simulink model "pendulumSystem"  (R2023b)
settings: Solver=VariableStepAuto  StartTime=0.0  StopTime=10.0  RelTol=1e-3
undefined symbols (not defined in the file or in its folder): X, Y, Z
libraries: sm_lib x8, nesl_utility x6, simulink_extras x3, fuzblock x2, slpidlib x2, simulink x1
settings Model: Creator=allef  LastModifiedBy=allef
settings SolverCC: ZeroCrossControl=DisableAll

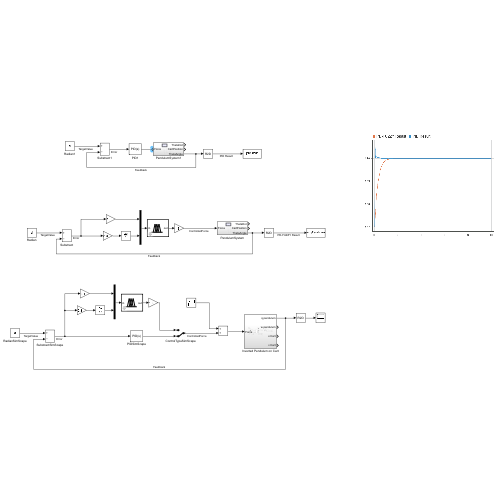
[thumbnail: Simulink's stored preview of the top-level diagram]
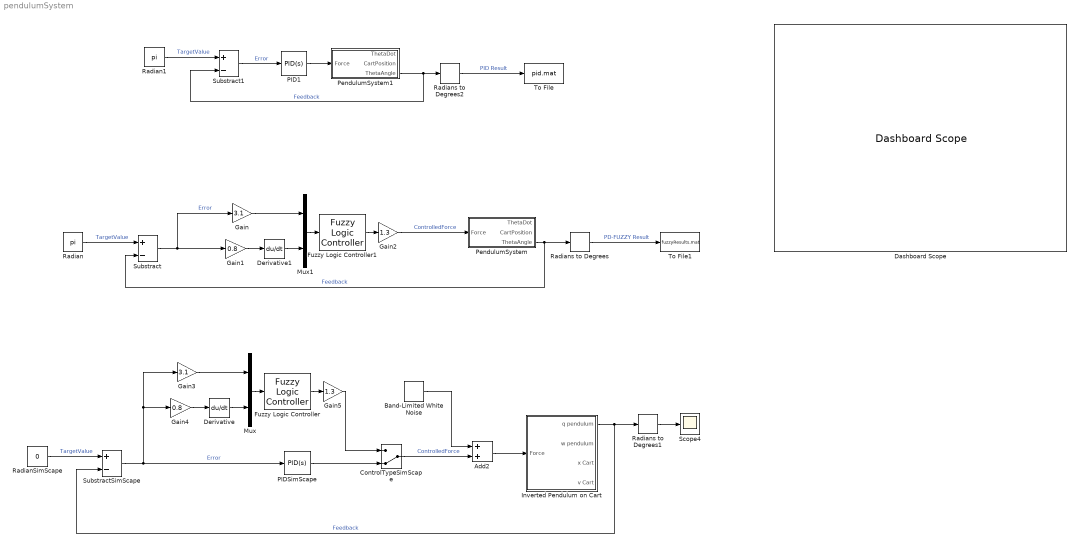
== system pendulumSystem ==
  Add2 : Sum
  Band-Limited White Noise : simulink/Sources/Band-Limited White Noise  Cov=[0.01]  Ts=0.1  seed=[23341]
  ControlTypeSimScape : ManualSwitch  CurrentSetting=0
  Dashboard Scope : DashboardScope
  Derivative : Derivative
  Derivative1 : Derivative
  Fuzzy Logic Controller : fuzblock/Fuzzy Logic  Controller  FIS='Fuzzy.fis'  OutputSampleNumber=101  DataType=double  FuzzifiedInputs=off  RuleFiringStrengths=off  RuleOutputs=off  AggregatedOutputs=off  SimulateUsing=Interpreted execution  OutOfRangeInputValueMessage=warning  NoRuleFiredMessage=warning  EmptyOutputFuzzySetMessage=warning
  Fuzzy Logic Controller1 : fuzblock/Fuzzy Logic  Controller  FIS='Fuzzy.fis'  OutputSampleNumber=101  DataType=double  FuzzifiedInputs=off  RuleFiringStrengths=off  RuleOutputs=off  AggregatedOutputs=off  SimulateUsing=Interpreted execution  OutOfRangeInputValueMessage=warning  NoRuleFiredMessage=warning  EmptyOutputFuzzySetMessage=warning
  Gain : Gain  Gain=3.1
  Gain1 : Gain  Gain=0.8
  Gain2 : Gain  Gain=1.3
  Gain3 : Gain  Gain=3.1
  Gain4 : Gain  Gain=0.8
  Gain5 : Gain  Gain=1.3
  Inverted Pendulum on Cart : Subsystem
  Mux : Mux  Inputs=2
  Mux1 : Mux  Inputs=2
  PID1 : slpidlib/PID Controller  Controller=PID  Form=Parallel  TimeDomain=Continuous-time  UseExternalTs=off  SampleTime=-1  IntegratorMethod=Forward Euler  FilterMethod=Forward Euler  ControllerParametersSource=internal  P=100  I=1  UseKiTs=off  D=20  N=100  UseFilter=on  TunerSelectOption=Transfer Function Based (PID Tuner App)  InitialConditionSource=internal  InitialConditionForIntegrator=0  InitialConditionForFilter=0  DifferentiatorICPrevScaledInput=0  ExternalReset=none  TrackingMode=off  Kt=1  LimitOutput=off  SatLimitsSource=internal  UpperSaturationLimit=inf  LowerSaturationLimit=-inf  LinearizeAsGain=on  AntiWindupMode=none  Kb=1  LimitIntegrator=off  UpperIntegratorSaturationLimit=inf  LowerIntegratorSaturationLimit=-inf  POutMin=[]  POutMax=[]  IOutMin=[]  IOutMax=[]  DOutMin=[]  DOutMax=[]  NOutMin=[]  NOutMax=[]  SumOutMin=[]  SumOutMax=[]  SaturationOutMin=[]  SaturationOutMax=[]  PParamMin=[]  PParamMax=[]  IParamMin=[]  IParamMax=[]  DParamMin=[]  DParamMax=[]  NParamMin=[]  NParamMax=[]  KbParamMin=[]  KbParamMax=[]  KtParamMin=[]  KtParamMax=[]  KbOutMin=[]  KbOutMax=[]  KtOutMin=[]  KtOutMax=[]  IntegratorOutMin=[]  IntegratorOutMax=[]  FilterOutMin=[]  FilterOutMax=[]  SumI1OutMin=[]  SumI1OutMax=[]  SumI2OutMin=[]  SumI2OutMax=[]  SumI3OutMin=[]  SumI3OutMax=[]  SumI4OutMin=[]  SumI4OutMax=[]  SumDOutMin=[]  SumDOutMax=[]  DifferentiatorOutMin=[]  DifferentiatorOutMax=[]  FilterDiffOutCoefMin=[]  FilterDiffOutCoefMax=[]  ReciprocalOutMin=[]  ReciprocalOutMax=[]  SumDenOutMin=[]  SumDenOutMax=[]  SumNumOutMin=[]  SumNumOutMax=[]  DivideOutMin=[]  DivideOutMax=[]  UdiffTsProdOutMin=[]  UdiffTsProdOutMax=[]  NTsProdOutMin=[]  NTsProdOutMax=[]  UintegralTsProdOutMin=[]  UintegralTsProdOutMax=[]  UngainTsProdOutMin=[]  UngainTsProdOutMax=[]  ClampingZeroOutDataTypeStr=Inherit: Inherit via back propagation  ClampingZeroOutMin=[]  ClampingZeroOutMax=[]  FilterDenConstantOutDataTypeStr=Inherit: Inherit via back propagation  FilterDenConstantOutMin=[]  FilterDenConstantOutMax=[]  PCopyOutDataTypeStr=Inherit: Inherit via back propagation  PCopyOutMin=[]  PCopyOutMax=[]  NCopyOutDataTypeStr=Inherit: Inherit via back propagation  NCopyOutMin=[]  NCopyOutMax=[]  IntegratorContinuousStateAttributes=''  IntegratorStateMustResolveToSignalObject=off  IntegratorRTWStateStorageClass=Auto  FilterContinuousStateAttributes=''  FilterStateMustResolveToSignalObject=off  FilterRTWStateStorageClass=Auto  ParallelPVariant=InternalParameters  IdealPVariant=Disabled  IVariant=InternalParameters  DVariant=InternalParameters  IntegratorVariant=Continuous  SatVariant=Disabled  AWVariant=Passthrough  PCopyVariant=Disabled  TRVariant=Disabled  FdbkBlocksVariant=Forward  IdealPFdbkVariant=Disabled  SatFdbkVariant=Disabled  DerivativeFilterVariant=ContFilter  NVariant=InternalParameters  NCopyVariant=Disabled  FilterICVariant=InternalICsFilter  IntegratorICVariant=InternalICs  ExternalResetVariant=Disabled  TRSumVariant=Passthrough  SumFdbkVariant=Disabled  SumVariant=Sum_PID  TsampFilterVariant=InternalTs  TsampNgainVariant=Passthrough  TsampIntegralVariant=Disabled_SignalSpec  ExternalSaturationOutDataTypeStr=Inherit: Same as second input
  PIDSimScape : slpidlib/PID Controller  Controller=PID  Form=Parallel  TimeDomain=Continuous-time  UseExternalTs=off  SampleTime=-1  IntegratorMethod=Forward Euler  FilterMethod=Forward Euler  ControllerParametersSource=internal  P=100  I=1  UseKiTs=off  D=20  N=100  UseFilter=on  TunerSelectOption=Transfer Function Based (PID Tuner App)  InitialConditionSource=internal  InitialConditionForIntegrator=0  InitialConditionForFilter=0  DifferentiatorICPrevScaledInput=0  ExternalReset=none  TrackingMode=off  Kt=1  LimitOutput=off  SatLimitsSource=internal  UpperSaturationLimit=inf  LowerSaturationLimit=-inf  LinearizeAsGain=on  AntiWindupMode=none  Kb=1  LimitIntegrator=off  UpperIntegratorSaturationLimit=inf  LowerIntegratorSaturationLimit=-inf  POutMin=[]  POutMax=[]  IOutMin=[]  IOutMax=[]  DOutMin=[]  DOutMax=[]  NOutMin=[]  NOutMax=[]  SumOutMin=[]  SumOutMax=[]  SaturationOutMin=[]  SaturationOutMax=[]  PParamMin=[]  PParamMax=[]  IParamMin=[]  IParamMax=[]  DParamMin=[]  DParamMax=[]  NParamMin=[]  NParamMax=[]  KbParamMin=[]  KbParamMax=[]  KtParamMin=[]  KtParamMax=[]  KbOutMin=[]  KbOutMax=[]  KtOutMin=[]  KtOutMax=[]  IntegratorOutMin=[]  IntegratorOutMax=[]  FilterOutMin=[]  FilterOutMax=[]  SumI1OutMin=[]  SumI1OutMax=[]  SumI2OutMin=[]  SumI2OutMax=[]  SumI3OutMin=[]  SumI3OutMax=[]  SumI4OutMin=[]  SumI4OutMax=[]  SumDOutMin=[]  SumDOutMax=[]  DifferentiatorOutMin=[]  DifferentiatorOutMax=[]  FilterDiffOutCoefMin=[]  FilterDiffOutCoefMax=[]  ReciprocalOutMin=[]  ReciprocalOutMax=[]  SumDenOutMin=[]  SumDenOutMax=[]  SumNumOutMin=[]  SumNumOutMax=[]  DivideOutMin=[]  DivideOutMax=[]  UdiffTsProdOutMin=[]  UdiffTsProdOutMax=[]  NTsProdOutMin=[]  NTsProdOutMax=[]  UintegralTsProdOutMin=[]  UintegralTsProdOutMax=[]  UngainTsProdOutMin=[]  UngainTsProdOutMax=[]  ClampingZeroOutDataTypeStr=Inherit: Inherit via back propagation  ClampingZeroOutMin=[]  ClampingZeroOutMax=[]  FilterDenConstantOutDataTypeStr=Inherit: Inherit via back propagation  FilterDenConstantOutMin=[]  FilterDenConstantOutMax=[]  PCopyOutDataTypeStr=Inherit: Inherit via back propagation  PCopyOutMin=[]  PCopyOutMax=[]  NCopyOutDataTypeStr=Inherit: Inherit via back propagation  NCopyOutMin=[]  NCopyOutMax=[]  IntegratorContinuousStateAttributes=''  IntegratorStateMustResolveToSignalObject=off  IntegratorRTWStateStorageClass=Auto  FilterContinuousStateAttributes=''  FilterStateMustResolveToSignalObject=off  FilterRTWStateStorageClass=Auto  ParallelPVariant=InternalParameters  IdealPVariant=Disabled  IVariant=InternalParameters  DVariant=InternalParameters  IntegratorVariant=Continuous  SatVariant=Disabled  AWVariant=Passthrough  PCopyVariant=Disabled  TRVariant=Disabled  FdbkBlocksVariant=Forward  IdealPFdbkVariant=Disabled  SatFdbkVariant=Disabled  DerivativeFilterVariant=ContFilter  NVariant=InternalParameters  NCopyVariant=Disabled  FilterICVariant=InternalICsFilter  IntegratorICVariant=InternalICs  ExternalResetVariant=Disabled  TRSumVariant=Passthrough  SumFdbkVariant=Disabled  SumVariant=Sum_PID  TsampFilterVariant=InternalTs  TsampNgainVariant=Passthrough  TsampIntegralVariant=Disabled_SignalSpec  ExternalSaturationOutDataTypeStr=Inherit: Same as second input
  PendulumSystem : Subsystem
  PendulumSystem1 : Subsystem
  Radian : Constant  Value=pi
  Radian1 : Constant  Value=pi
  RadianSimScape : Constant  Value=0
  Radians to Degrees : simulink_extras/Transformations/Radians to Degrees
  Radians to Degrees1 : simulink_extras/Transformations/Radians to Degrees
  Radians to Degrees2 : simulink_extras/Transformations/Radians to Degrees
  Scope4 : Scope
  Substract : Sum  Inputs=+-
  Substract1 : Sum  Inputs=+-
  SubstractSimScape : Sum  Inputs=+-
  To File : ToFile  Filename=pid.mat  MatrixName=pid
  To File1 : ToFile  Filename=fuzzyResults.mat  MatrixName=fuzzy
  wires:
  Substract/1 -> Gain/1, Gain1/1  "Error"
  Radian/1 -> Substract/1  "TargetValue"
  PendulumSystem/3(ThetaAngle) -> Substract/2, Radians to Degrees/1  "Feedback"
  Radians to Degrees/1 -> To File1/1  "PD-FUZZY Result"
  ControlTypeSimScape/1 -> Add2/2  "ControlledForce"
  RadianSimScape/1 -> SubstractSimScape/1  "TargetValue"
  SubstractSimScape/1 -> PIDSimScape/1, Gain4/1, Gain3/1  "Error"
  PIDSimScape/1 -> ControlTypeSimScape/2
  Derivative/1 -> Mux/2
  Mux/1 -> Fuzzy Logic Controller/1
  Fuzzy Logic Controller/1 -> Gain5/1
  Derivative1/1 -> Mux1/2
  Mux1/1 -> Fuzzy Logic Controller1/1
  Fuzzy Logic Controller1/1 -> Gain2/1
  Gain/1 -> Mux1/1
  Gain1/1 -> Derivative1/1
  Gain3/1 -> Mux/1
  Gain4/1 -> Derivative/1
  Gain5/1 -> ControlTypeSimScape/1
  Add2/1 -> Inverted Pendulum on Cart/1(Force)
  Inverted Pendulum on Cart/1(q pendulum) -> SubstractSimScape/2, Radians to Degrees1/1  "Feedback"
  Radians to Degrees1/1 -> Scope4/1
  Gain2/1 -> PendulumSystem/1(Force)  "ControlledForce"
  Band-Limited White Noise/1 -> Add2/1
  Radians to Degrees2/1 -> To File/1  "PID Result"
  PendulumSystem1/3(ThetaAngle) -> Radians to Degrees2/1, Substract1/2  "Feedback"
  PID1/1 -> PendulumSystem1/1(Force)
  Radian1/1 -> Substract1/1  "TargetValue"
  Substract1/1 -> PID1/1  "Error"

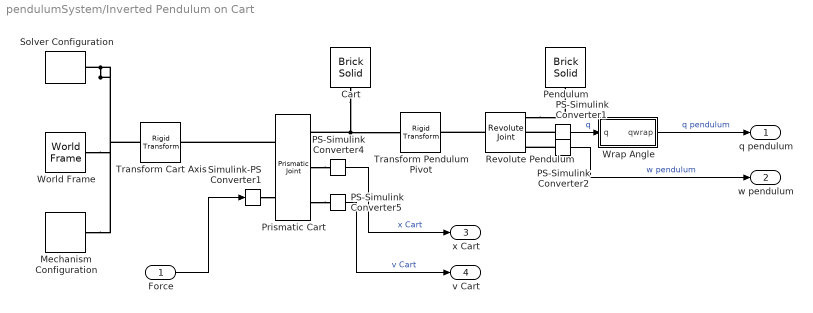
== system pendulumSystem/Inverted Pendulum on Cart ==
  Force : Inport
  Cart : sm_lib/Body Elements/Brick Solid  GraphicAmbientColor=[0.15 0.15 0.15 1.0]  BasedOnType=Density  BrickDimensions=[0.2 0.04 .60]  BrickDimensionsUnits=m  CenterOfMass=[0 0 0]  CenterOfMassUnits=m  GraphicDiffuseColor=[0.8 0.45 0]  Density=1000  DensityUnits=kg/m^3  DoExposeReferenceFrame=on  GraphicEmissiveColor=[0.0 0.0 0.0 1.0]  ExportEntireGeometry=off  SerializedFrames=<Frames/>  MarkerShape=Sphere  MarkerSize=10  GraphicType=FromGeometry  InertiaType=PointMass  Mass=0.5  MassUnits=kg  MomentsOfInertia=[1 1 1]  MomentsOfInertiaUnits=kg*m^2  GraphicOpacity=1.0  ProductsOfInertia=[0 0 0]  ProductsOfInertiaUnits=kg*m^2  GraphicShininess=75  GraphicSpecularColor=[0.5 0.5 0.5 1.0]  GraphicVisPropType=SimpleVisualProperties
  Mechanism Configuration : sm_lib/Utilities/Mechanism Configuration  UniformGravity=Constant  GravityVector=[0 0 -9.80665]  GravityVectorUnits=m/s^2  LinearizationDelta=0.001  JointModeTransitionNonlinearIterations=2
  PS-Simulink Converter1 : nesl_utility/PS-Simulink Converter  PhysicalDomain=network_engine_domain  SubClassName=ps_output  LeftPortType=input  RightPortType=output  PseudoPeriodic=off  Frequencies=[]  VectorFormat=1-D array  Unit=rad  AffineConversion=off
  PS-Simulink Converter2 : nesl_utility/PS-Simulink Converter  PhysicalDomain=network_engine_domain  SubClassName=ps_output  LeftPortType=input  RightPortType=output  PseudoPeriodic=off  Frequencies=[]  VectorFormat=1-D array  Unit=rad/s  AffineConversion=off
  PS-Simulink Converter4 : nesl_utility/PS-Simulink Converter  PhysicalDomain=network_engine_domain  SubClassName=ps_output  LeftPortType=input  RightPortType=output  PseudoPeriodic=off  Frequencies=[]  VectorFormat=1-D array  Unit=m  AffineConversion=off
  PS-Simulink Converter5 : nesl_utility/PS-Simulink Converter  PhysicalDomain=network_engine_domain  SubClassName=ps_output  LeftPortType=input  RightPortType=output  PseudoPeriodic=off  Frequencies=[]  VectorFormat=1-D array  Unit=m/s  AffineConversion=off
  Pendulum : sm_lib/Body Elements/Brick Solid  GraphicAmbientColor=[0.15 0.15 0.15 1.0]  BasedOnType=Density  BrickDimensions=[0.6 0.03 0.05]  BrickDimensionsUnits=m  CenterOfMass=[0 0 0]  CenterOfMassUnits=m  GraphicDiffuseColor=[0.25 0.4 0.7]  Density=1000  DensityUnits=kg/m^3  DoExposeReferenceFrame=off  GraphicEmissiveColor=[0.0 0.0 0.0 1.0]  ExportEntireGeometry=off  SerializedFrames=<Frames><Frame><Id>Frame1</Id><Value><Name>B</Name><Origin><Source>GeometricFeature</Source><FeatureName>+x surface</FeatureName></Origin><PrimaryAxis><DefinedDirection>+Z</DefinedDirection><Source>ReferenceFrame</Source><SourceDirection>+Z</SourceDirection><FeatureName></FeatureName></PrimaryAxis><SecondaryAxis><DefinedDirection>+X</DefinedDirection><Source>ReferenceFrame</Source><SourceDirection>+X</SourceDirection><FeatureName></FeatureName></SecondaryAxis></Value></Frame></Frames>  MarkerShape=Sphere  MarkerSize=10  GraphicType=FromGeometry  InertiaType=PointMass  Mass=0.2  MassUnits=kg  MomentsOfInertia=[1 1 1]  MomentsOfInertiaUnits=kg*m^2  GraphicOpacity=1.0  ProductsOfInertia=[0 0 0]  ProductsOfInertiaUnits=kg*m^2  GraphicShininess=75  GraphicSpecularColor=[0.5 0.5 0.5 1.0]  GraphicVisPropType=SimpleVisualProperties
  Prismatic Cart : sm_lib/Joints/Prismatic Joint  JointMode=Normal  SenseConstraintForce=off  SenseConstraintForceX=off  SenseConstraintForceY=off  SenseConstraintForceZ=off  SenseConstraintTorque=off  SenseConstraintTorqueX=off  SenseConstraintTorqueY=off  SenseConstraintTorqueZ=off  SenseTotalForce=off  SenseTotalForceX=off  SenseTotalForceY=off  SenseTotalForceZ=off  SenseTotalTorque=off  SenseTotalTorqueX=off  SenseTotalTorqueY=off  SenseTotalTorqueZ=off  CompositeWrenchDir=FollowerOnBase  CompositeWrenchFrame=BaseFrame  EquilibriumPosition=0  EquilibriumPositionUnits=m  SpringStiffness=0  SpringStiffnessUnits=N/m  DampingCoefficient=0.1  DampingCoefficientUnits=N/(m/s)  TorqueActuationMode=InputTorque  MotionActuationMode=ComputedMotion  SensePosition=on  SenseVelocity=on  SenseAcceleration=off  SenseTorqueForce=off  SenseLowerLimitTorqueForce=off  SenseUpperLimitTorqueForce=off  LowerLimitSpecify=off  LowerLimitBound=-1  LowerLimitBoundUnits=m  LowerLimitStiffness=1e6  LowerLimitStiffnessUnits=N/m  LowerLimitDamping=1e3  LowerLimitDampingUnits=N/(m/s)  LowerLimitTransitionRegionWidth=1e-4  LowerLimitTransitionRegionWidthUnits=m  UpperLimitSpecify=off  UpperLimitBound=1  UpperLimitBoundUnits=m  UpperLimitStiffness=1e6  UpperLimitStiffnessUnits=N/m  UpperLimitDamping=1e3  UpperLimitDampingUnits=N/(m/s)  UpperLimitTransitionRegionWidth=1e-4  UpperLimitTransitionRegionWidthUnits=m  PositionTargetSpecify=off  PositionTargetPriority=High  PositionTargetValue=0  PositionTargetValueUnits=m  VelocityTargetSpecify=off  VelocityTargetPriority=High  VelocityTargetValue=0  VelocityTargetValueUnits=m/s
  Revolute Pendulum : sm_lib/Joints/Revolute Joint  JointMode=Normal  SenseConstraintForce=off  SenseConstraintForceX=off  SenseConstraintForceY=off  SenseConstraintForceZ=off  SenseConstraintTorque=off  SenseConstraintTorqueX=off  SenseConstraintTorqueY=off  SenseConstraintTorqueZ=off  SenseTotalForce=off  SenseTotalForceX=off  SenseTotalForceY=off  SenseTotalForceZ=off  SenseTotalTorque=off  SenseTotalTorqueX=off  SenseTotalTorqueY=off  SenseTotalTorqueZ=off  CompositeWrenchDir=FollowerOnBase  CompositeWrenchFrame=BaseFrame  EquilibriumPosition=0  EquilibriumPositionUnits=deg  SpringStiffness=0  SpringStiffnessUnits=N*m/deg  DampingCoefficient=0  DampingCoefficientUnits=N*m/(deg/s)  TorqueActuationMode=NoTorque  MotionActuationMode=ComputedMotion  SensePosition=on  SenseVelocity=on  SenseAcceleration=off  SenseTorqueForce=off  SenseLowerLimitTorqueForce=off  SenseUpperLimitTorqueForce=off  LowerLimitSpecify=off  LowerLimitBound=-90  LowerLimitBoundUnits=deg  LowerLimitStiffness=1e4  LowerLimitStiffnessUnits=N*m/deg  LowerLimitDamping=10  LowerLimitDampingUnits=N*m/(deg/s)  LowerLimitTransitionRegionWidth=0.1  LowerLimitTransitionRegionWidthUnits=deg  UpperLimitSpecify=off  UpperLimitBound=90  UpperLimitBoundUnits=deg  UpperLimitStiffness=1e4  UpperLimitStiffnessUnits=N*m/deg  UpperLimitDamping=10  UpperLimitDampingUnits=N*m/(deg/s)  UpperLimitTransitionRegionWidth=0.1  UpperLimitTransitionRegionWidthUnits=deg  PositionTargetSpecify=off  PositionTargetPriority=High  PositionTargetValue=0  PositionTargetValueUnits=deg  VelocityTargetSpecify=off  VelocityTargetPriority=High  VelocityTargetValue=0  VelocityTargetValueUnits=deg/s
  Simulink-PS Converter1 : nesl_utility/Simulink-PS Converter  PhysicalDomain=network_engine_domain  SubClassName=ps_input  LeftPortType=input  RightPortType=output  PseudoPeriodic=off  Frequencies=[]  NoiseDistribution=none  NoiseParameters=[]  Unit=N  AffineConversion=off  FilteringAndDerivatives=zero  SimscapeFilterOrder=1  InputFilterTimeConstant=.001  UdotUserProvided=1
  Solver Configuration : nesl_utility/Solver Configuration  PhysicalDomain=network_engine_domain  SubClassName=solver  LeftPortType=input  RightPortType=generic  Tones=[]  Harmonics=[]  SimulateNoise=off  Profile=off  UseLocalSampling=off  EnableSwitchedLinearOptims=on  FrequencyDomain=off  UseCCode=off  RelTol=0.001  AbsTol=1e-06  MinStep=1e-09  ToWorkspace=off  RevertToSquareIcSolve=off  NumHomotopyIterations=100  PhasorMode=off  PhasorModeNumHarmonics=1  ConsistencySolver=NEWTON_FTOL  IndexReductionMethod=DerivativeReplacement  DoDC=off  ResidualTolerance=1e-09  ConsistencyTolSource=GLOBAL  ConsistencyAbsTol=0.001  ConsistencyRelTol=0.001  ConsistencyTolFactor=0.001  UseLocalSolver=off  LocalSolverChoice=NE_BACKWARD_EULER_ADVANCER  ResolveIndetEquations=on  FunctionEvalNumThread=1  LocalSolverSampleTime=0.001  DoFixedCost=off  MaxNonlinIter=3  MaxModeIter=2  ComputeImpulses=off  ImpulseIterations=2  LinearAlgebra=Sparse  LinearAlgebraNumThread=0  EquationFormulation=NE_TIME_EF  DelaysMemoryBudget=1024  AutomaticFiltering=on  FilteringTimeConstant=0.001  PartitionStorageMethod=AS_NEEDED  PartitionMemoryBudget=1024  PartitionMethod=FAST  MultibodyUseLocalSolver=off  MultibodyLocalSolverChoice=ODE1  MultibodyLocalSolverSampleTime=0.001
  Transform Cart Axis : sm_lib/Frames and Transforms/Rigid Transform  TranslationMethod=None  TranslationStandardOffset=0  TranslationStandardOffsetUnits=m  TranslationStandardAxis=+Z  TranslationCartesianOffset=[0 0 0]  TranslationCartesianOffsetUnits=m  TranslationROffset=0  TranslationROffsetUnits=m  TranslationZOffset=0  TranslationZOffsetUnits=m  TranslationThetaOffset=0  TranslationThetaOffsetUnits=deg  RotationMethod=StandardAxis  RotationAngleUnits=deg  RotationStandardAxis=+Y  RotationAngle=90  RotationArbitraryAxis=[0 0 1]  FollAlignAxisA=+X  BaseAlignAxisA=+Y  FollAlignAxisB=+Y  BaseAlignAxisB=+Z  RotationSequenceAxes=FollowerAxes  RotationSequence=XYX  RotationSequenceAngles=[0 0 0]  RotationSequenceAnglesUnits=deg  RotationMatrix=[1 0 0; 0 1 0; 0 0 1]  Quaternion=[1 0 0 0]
  Transform Pendulum Pivot : sm_lib/Frames and Transforms/Rigid Transform  TranslationMethod=None  TranslationStandardOffset=0.025  TranslationStandardOffsetUnits=m  TranslationStandardAxis=-X  TranslationCartesianOffset=[0 0 0]  TranslationCartesianOffsetUnits=m  TranslationROffset=0  TranslationROffsetUnits=m  TranslationZOffset=0  TranslationZOffsetUnits=m  TranslationThetaOffset=0  TranslationThetaOffsetUnits=deg  RotationMethod=StandardAxis  RotationAngleUnits=deg  RotationStandardAxis=+X  RotationAngle=90  RotationArbitraryAxis=[0 0 1]  FollAlignAxisA=+X  BaseAlignAxisA=+Y  FollAlignAxisB=+Y  BaseAlignAxisB=+Z  RotationSequenceAxes=FollowerAxes  RotationSequence=XYX  RotationSequenceAngles=[0 0 0]  RotationSequenceAnglesUnits=deg  RotationMatrix=[1 0 0; 0 1 0; 0 0 1]  Quaternion=[1 0 0 0]
  World Frame : sm_lib/Frames and Transforms/World Frame
  Wrap Angle : Subsystem
  q pendulum : Outport  VectorParamsAs1DForOutWhenUnconnected=off
  w pendulum : Outport  Port=2  VectorParamsAs1DForOutWhenUnconnected=off
  x Cart : Outport  Port=3  VectorParamsAs1DForOutWhenUnconnected=off
  v Cart : Outport  Port=4  VectorParamsAs1DForOutWhenUnconnected=off
  wires:
  PS-Simulink Converter1/1 -> Wrap Angle/1(q)  "q"
  Force/1 -> Simulink-PS Converter1/1
  PS-Simulink Converter4/1 -> x Cart/1  "x Cart"
  PS-Simulink Converter5/1 -> v Cart/1  "v Cart"
  PS-Simulink Converter2/1 -> w pendulum/1  "w pendulum"
  Wrap Angle/1(qwrap) -> q pendulum/1  "q pendulum"
  connections:
  Revolute Pendulum/LConn1 -- Transform Pendulum Pivot/RConn1
  Solver Configuration/RConn1 -- Mechanism Configuration/RConn1 -- World Frame/RConn1 -- Transform Cart Axis/LConn1
  Prismatic Cart/RConn2 -- PS-Simulink Converter4/LConn1
  PS-Simulink Converter1/LConn1 -- Revolute Pendulum/RConn2
  Revolute Pendulum/RConn1 -- Pendulum/LConn1
  Cart/RConn1 -- Prismatic Cart/RConn1 -- Transform Pendulum Pivot/LConn1
  Prismatic Cart/RConn3 -- PS-Simulink Converter5/LConn1
  PS-Simulink Converter2/LConn1 -- Revolute Pendulum/RConn3
  Prismatic Cart/LConn1 -- Transform Cart Axis/RConn1
  Simulink-PS Converter1/RConn1 -- Prismatic Cart/LConn2

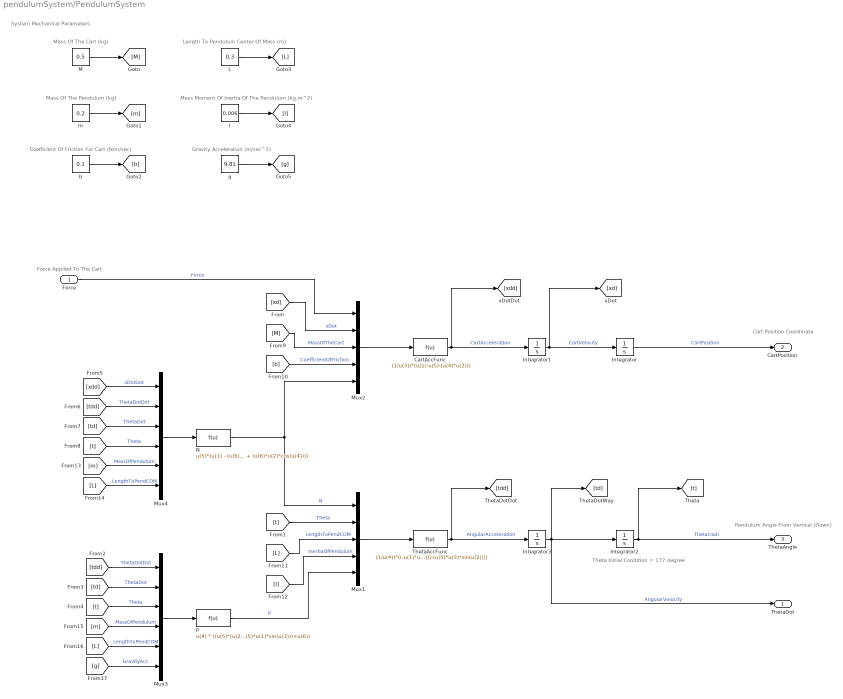
== system pendulumSystem/PendulumSystem ==
  note: Theta Initial Condition = 177 degree
  note: System Mechanical Parameters
  note: Force Applied To The Cart
  note: Cart Position Coordinate
  note: Pendulum Angle From Vertical (Down)
  note: Mass Moment Of Inertia Of The Pendulum (kg.m^2)
  note: Length To Pendulum Center Of Mass (m)
  note: Coefficient Of Friction For Cart (N/m/sec)
  note: Mass Of The Pendulum (kg)
  note: Mass Of The Cart (kg)
  note: Gravity Acceleration (m/sec^2)
  Force : Inport
  CartAccFunc : Fcn  Expr=(1/u(3))*(u(1)-u(5)-(u(4)*u(2)))
  I : Constant  Value=0.006
  Integrator : Integrator
  Integrator1 : Integrator
  Integrator2 : Integrator  InitialCondition=pi-0.05235987755983
  Integrator3 : Integrator
  L : Constant  Value=0.3
  M : Constant  Value=0.5
  Mux1 : Mux  Inputs=5
  Mux2 : Mux  Inputs=5
  Mux3 : Mux  Inputs=6
  Mux4 : Mux  Inputs=6
  N : Fcn  Expr=u(5)*(u(1) - (u(6)*(u(3)^2)*sin(u(4))) + (u(6)*u(2)*cos(u(4))))
  P : Fcn  Expr=u(4) * ((u(5)*(u(2)^2)*cos(u(3)))+(u(5)*u(1)*sin(u(3)))+u(6))
  ThetaAccFunc : Fcn  Expr=(1/u(4))*((-u(1)*u(3)*cos(u(2)))-(u(5)*u(3)*sin(u(2))))
  b : Constant  Value=0.1
  g : Constant  Value=9.81
  m : Constant  Value=0.2
  ThetaDot : Outport
  CartPosition : Outport  Port=2
  ThetaAngle : Outport  Port=3
  wires:
  Integrator/1 -> CartPosition/1  "CartPosition"
  Integrator1/1 -> [xd], Integrator/1  "CartVelocity"
  Integrator3/1 -> ThetaDot/1, [td], Integrator2/1  "AngularVelocity"
  Integrator2/1 -> ThetaAngle/1, [t]  "Theta(rad)"
  ThetaAccFunc/1 -> [tdd], Integrator3/1  "AngularAcceleration"
  CartAccFunc/1 -> [xdd], Integrator1/1  "CartAcceleration"
  Mux2/1 -> CartAccFunc/1
  Mux1/1 -> ThetaAccFunc/1
  M/1 -> [M]
  m/1 -> [m]
  b/1 -> [b]
  L/1 -> [L]
  I/1 -> [I]
  Force/1 -> Mux2/1  "Force"
  [xd] -> Mux2/2  "xDot"
  [t] -> Mux1/2  "Theta"
  N/1 -> Mux1/1, Mux2/5  "N"
  Mux3/1 -> P/1
  Mux4/1 -> N/1
  [xdd] -> Mux4/1  "xDotDot"
  [tdd] -> Mux4/2  "ThetaDotDot"
  [td] -> Mux4/3  "ThetaDot"
  [t] -> Mux4/4  "Theta"
  [M] -> Mux2/3  "MassOfTheCart"
  [b] -> Mux2/4  "CoefficientOfFriction"
  P/1 -> Mux1/5  "P"
  [L] -> Mux1/3  "LengthToPendCOM"
  [I] -> Mux1/4  "InertiaOfPendulum"
  [m] -> Mux4/5  "MassOfPendulum"
  [L] -> Mux4/6  "LengthToPendCOM"
  g/1 -> [g]
  [tdd] -> Mux3/1  "ThetaDotDot"
  [td] -> Mux3/2  "ThetaDot"
  [t] -> Mux3/3  "Theta"
  [m] -> Mux3/4  "MassOfPendulum"
  [L] -> Mux3/5  "LengthToPendCOM"
  [g] -> Mux3/6  "GravityAcc"

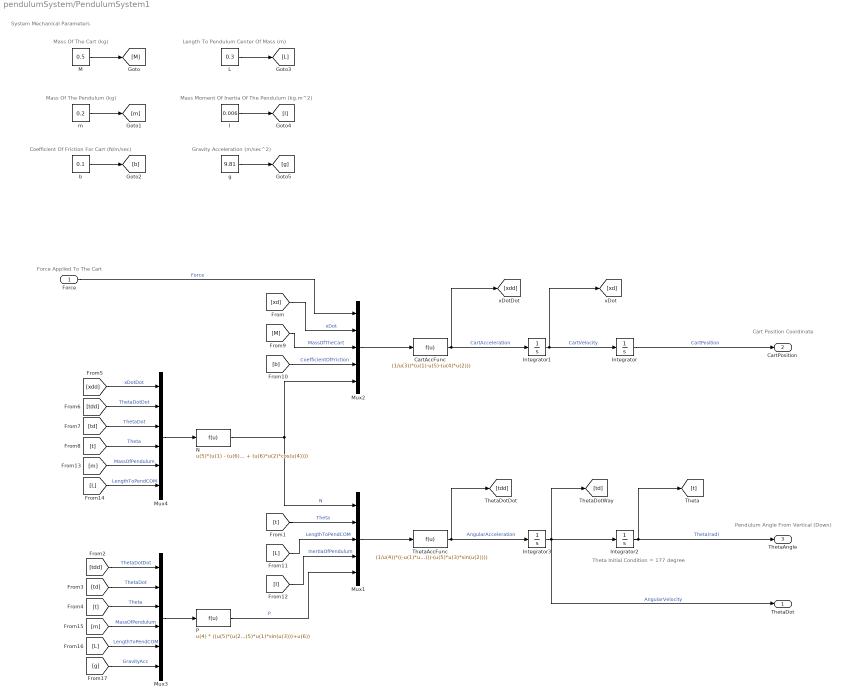
== system pendulumSystem/PendulumSystem1 ==
  note: Gravity Acceleration (m/sec^2)
  note: Mass Of The Cart (kg)
  note: Mass Of The Pendulum (kg)
  note: Coefficient Of Friction For Cart (N/m/sec)
  note: Length To Pendulum Center Of Mass (m)
  note: Mass Moment Of Inertia Of The Pendulum (kg.m^2)
  note: Pendulum Angle From Vertical (Down)
  note: Cart Position Coordinate
  note: Force Applied To The Cart
  note: System Mechanical Parameters
  note: Theta Initial Condition = 177 degree
  Force : Inport
  CartAccFunc : Fcn  Expr=(1/u(3))*(u(1)-u(5)-(u(4)*u(2)))
  I : Constant  Value=0.006
  Integrator : Integrator
  Integrator1 : Integrator
  Integrator2 : Integrator  InitialCondition=pi-0.05235987755983
  Integrator3 : Integrator
  L : Constant  Value=0.3
  M : Constant  Value=0.5
  Mux1 : Mux  Inputs=5
  Mux2 : Mux  Inputs=5
  Mux3 : Mux  Inputs=6
  Mux4 : Mux  Inputs=6
  N : Fcn  Expr=u(5)*(u(1) - (u(6)*(u(3)^2)*sin(u(4))) + (u(6)*u(2)*cos(u(4))))
  P : Fcn  Expr=u(4) * ((u(5)*(u(2)^2)*cos(u(3)))+(u(5)*u(1)*sin(u(3)))+u(6))
  ThetaAccFunc : Fcn  Expr=(1/u(4))*((-u(1)*u(3)*cos(u(2)))-(u(5)*u(3)*sin(u(2))))
  b : Constant  Value=0.1
  g : Constant  Value=9.81
  m : Constant  Value=0.2
  ThetaDot : Outport
  CartPosition : Outport  Port=2
  ThetaAngle : Outport  Port=3
  wires:
  [g] -> Mux3/6  "GravityAcc"
  [L] -> Mux3/5  "LengthToPendCOM"
  [m] -> Mux3/4  "MassOfPendulum"
  [t] -> Mux3/3  "Theta"
  [td] -> Mux3/2  "ThetaDot"
  [tdd] -> Mux3/1  "ThetaDotDot"
  g/1 -> [g]
  [L] -> Mux4/6  "LengthToPendCOM"
  [m] -> Mux4/5  "MassOfPendulum"
  [I] -> Mux1/4  "InertiaOfPendulum"
  [L] -> Mux1/3  "LengthToPendCOM"
  P/1 -> Mux1/5  "P"
  [b] -> Mux2/4  "CoefficientOfFriction"
  [M] -> Mux2/3  "MassOfTheCart"
  [t] -> Mux4/4  "Theta"
  [td] -> Mux4/3  "ThetaDot"
  [tdd] -> Mux4/2  "ThetaDotDot"
  [xdd] -> Mux4/1  "xDotDot"
  Mux4/1 -> N/1
  Mux3/1 -> P/1
  N/1 -> Mux2/5, Mux1/1  "N"
  [t] -> Mux1/2  "Theta"
  [xd] -> Mux2/2  "xDot"
  Force/1 -> Mux2/1  "Force"
  I/1 -> [I]
  L/1 -> [L]
  b/1 -> [b]
  m/1 -> [m]
  M/1 -> [M]
  Mux1/1 -> ThetaAccFunc/1
  Mux2/1 -> CartAccFunc/1
  CartAccFunc/1 -> Integrator1/1, [xdd]  "CartAcceleration"
  ThetaAccFunc/1 -> Integrator3/1, [tdd]  "AngularAcceleration"
  Integrator2/1 -> [t], ThetaAngle/1  "Theta(rad)"
  Integrator3/1 -> Integrator2/1, [td], ThetaDot/1  "AngularVelocity"
  Integrator1/1 -> Integrator/1, [xd]  "CartVelocity"
  Integrator/1 -> CartPosition/1  "CartPosition"

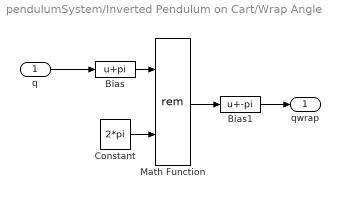
== system pendulumSystem/Inverted Pendulum on Cart/Wrap Angle ==
  q : Inport
  Bias : Bias  Bias=pi  SaturateOnIntegerOverflow=off
  Bias1 : Bias  Bias=-pi  SaturateOnIntegerOverflow=off
  Constant : Constant  Value=2*pi
  Math Function : Math  Operator=rem  SignedPower=on
  qwrap : Outport  VectorParamsAs1DForOutWhenUnconnected=off
  wires:
  q/1 -> Bias/1
  Constant/1 -> Math Function/2
  Math Function/1 -> Bias1/1
  Bias/1 -> Math Function/1
  Bias1/1 -> qwrap/1
